simulink model "motor_model"  (R2018b)
settings: Solver=VariableStepAuto  StartTime=0.0  StopTime=2  RelTol=1e-3
model workspace (MAT data in the model file):
  Ce = 0.1
  Cm = 0.1
  Jsumm = 0.00025
  Kf = 0.1
  L = 0.0001
  R = 0.52
  U = 13.5
  poles = 8
libraries: simulink x2
settings Model: Creator=Sainquake  LastModifiedBy=Sainquake

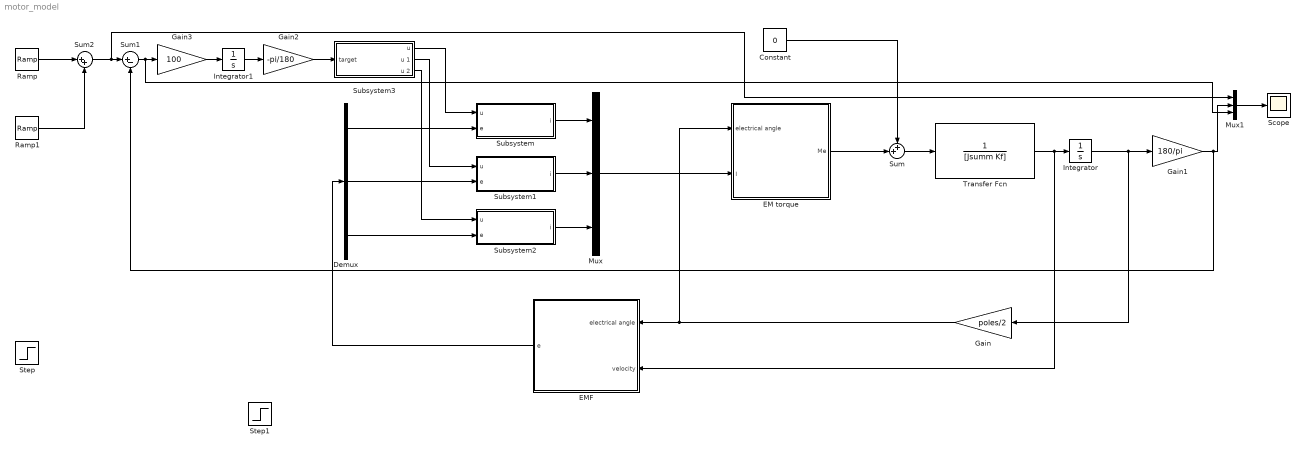
== system motor_model ==
  Constant : Constant  Value=0
  Demux : Demux  Outputs=3
  EM torque : Subsystem
  EMF : Subsystem
  Gain : Gain  Gain=poles/2
  Gain1 : Gain  Gain=180/pi
  Gain2 : Gain  Gain=-pi/180
  Gain3 : Gain  Gain=100
  Integrator : Integrator
  Integrator1 : Integrator
  Mux : Mux  Inputs=3
  Mux1 : Mux  Inputs=3
  Ramp : simulink/Sources/Ramp  slope=90/0.6  start=0  InitialOutput=0
  Ramp1 : simulink/Sources/Ramp  slope=-90/0.6  start=0.6  InitialOutput=0
  Scope : Scope
  Step : Step  Time=10  After=10  SampleTime=0
  Step1 : Step  SampleTime=0
  Subsystem : Subsystem
  Subsystem1 : Subsystem
  Subsystem2 : Subsystem
  Subsystem3 : Subsystem
  Sum : Sum  Inputs=++|
  Sum1 : Sum  Inputs=|+-
  Sum2 : Sum  Inputs=|++
  Transfer Fcn : TransferFcn  Denominator=[Jsumm Kf]
  wires:
  Subsystem/1(i) -> Mux/1
  Subsystem2/1(i) -> Mux/3
  Subsystem1/1(i) -> Mux/2
  Mux/1 -> EM torque/2(I)
  Demux/1 -> Subsystem/2("e ")
  Demux/2 -> Subsystem1/2("e ")
  Demux/3 -> Subsystem2/2("e ")
  EMF/1(e) -> Demux/1
  EM torque/1(Me) -> Sum/2
  Constant/1 -> Sum/1
  Sum/1 -> Transfer Fcn/1
  Transfer Fcn/1 -> EMF/2(velocity), Integrator/1
  Integrator/1 -> Gain1/1, Gain/1
  Gain/1 -> EM torque/1(electrical angle), EMF/1(electrical angle)
  Subsystem3/1("u ") -> Subsystem/1(u)
  Subsystem3/2(u 1) -> Subsystem1/1(u)
  Subsystem3/3(u 2) -> Subsystem2/1(u)
  Gain2/1 -> Subsystem3/1(target)
  Mux1/1 -> Scope/1
  Gain1/1 -> Mux1/2, Sum1/2
  Sum2/1 -> Mux1/1, Sum1/1
  Integrator1/1 -> Gain2/1
  Gain3/1 -> Integrator1/1
  Ramp/1 -> Sum2/1
  Ramp1/1 -> Sum2/2
  Sum1/1 -> Mux1/3, Gain3/1

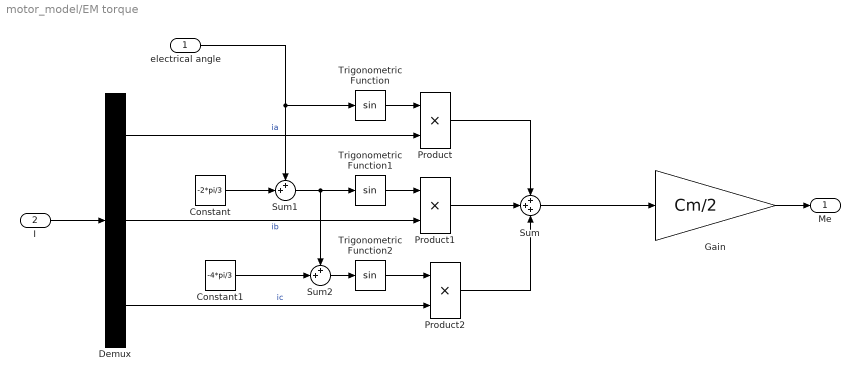
== system motor_model/EM torque ==
  electrical angle : Inport
  I : Inport  Port=2
  Constant : Constant  Value=-2*pi/3
  Constant1 : Constant  Value=-4*pi/3
  Demux : Demux  Outputs=3
  Gain : Gain  Gain=Cm/2
  Product : Product
  Product1 : Product
  Product2 : Product
  Sum : Sum  Inputs=+++
  Sum1 : Sum  Inputs=++|
  Sum2 : Sum  Inputs=++|
  Trigonometric Function : Trigonometry
  Trigonometric Function1 : Trigonometry
  Trigonometric Function2 : Trigonometry
  Me : Outport
  wires:
  Trigonometric Function/1 -> Product/1
  Product/1 -> Sum/1
  Sum/1 -> Gain/1
  Gain/1 -> Me/1
  Demux/1 -> Product/2  "ia"
  Trigonometric Function1/1 -> Product1/1
  Demux/2 -> Product1/2  "ib"
  Trigonometric Function2/1 -> Product2/1
  Demux/3 -> Product2/2  "ic"
  Product2/1 -> Sum/3
  Product1/1 -> Sum/2
  I/1 -> Demux/1
  Sum1/1 -> Sum2/1, Trigonometric Function1/1
  Constant/1 -> Sum1/2
  electrical angle/1 -> Trigonometric Function/1, Sum1/1
  Constant1/1 -> Sum2/2
  Sum2/1 -> Trigonometric Function2/1

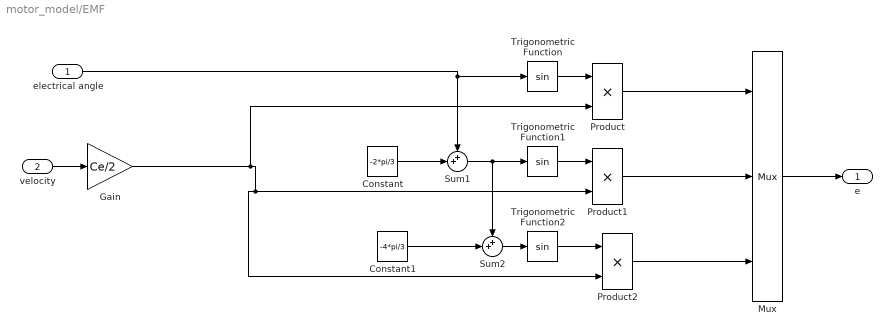
== system motor_model/EMF ==
  electrical angle : Inport
  velocity : Inport  Port=2
  Constant : Constant  Value=-2*pi/3
  Constant1 : Constant  Value=-4*pi/3
  Gain : Gain  Gain=Ce/2
  Mux : Mux  Inputs=3
  Product : Product
  Product1 : Product
  Product2 : Product
  Sum1 : Sum  Inputs=++|
  Sum2 : Sum  Inputs=++|
  Trigonometric Function : Trigonometry
  Trigonometric Function1 : Trigonometry
  Trigonometric Function2 : Trigonometry
  e : Outport
  wires:
  Trigonometric Function/1 -> Product/1
  Trigonometric Function1/1 -> Product1/1
  Trigonometric Function2/1 -> Product2/1
  Gain/1 -> Product2/2, Product1/2, Product/2
  Sum1/1 -> Sum2/1, Trigonometric Function1/1
  Constant/1 -> Sum1/2
  electrical angle/1 -> Trigonometric Function/1, Sum1/1
  Constant1/1 -> Sum2/2
  Sum2/1 -> Trigonometric Function2/1
  Mux/1 -> e/1
  velocity/1 -> Gain/1
  Product/1 -> Mux/1
  Product1/1 -> Mux/2
  Product2/1 -> Mux/3

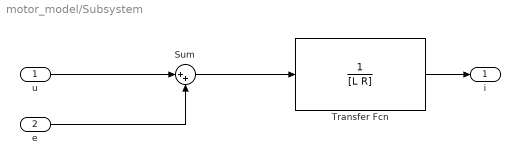
== system motor_model/Subsystem ==
  u : Inport
  "e " : Inport  Port=2
  Sum : Sum  Inputs=|++
  Transfer Fcn : TransferFcn  Denominator=[L R]
  i : Outport
  wires:
  u/1 -> Sum/1
  Transfer Fcn/1 -> i/1
  Sum/1 -> Transfer Fcn/1
  "e "/1 -> Sum/2

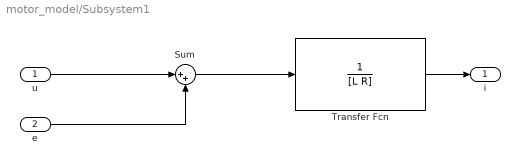
== system motor_model/Subsystem1 ==
  u : Inport
  "e " : Inport  Port=2
  Sum : Sum  Inputs=|++
  Transfer Fcn : TransferFcn  Denominator=[L R]
  i : Outport
  wires:
  u/1 -> Sum/1
  Transfer Fcn/1 -> i/1
  Sum/1 -> Transfer Fcn/1
  "e "/1 -> Sum/2

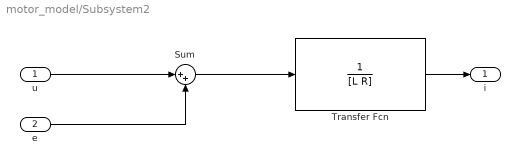
== system motor_model/Subsystem2 ==
  u : Inport
  "e " : Inport  Port=2
  Sum : Sum  Inputs=|++
  Transfer Fcn : TransferFcn  Denominator=[L R]
  i : Outport
  wires:
  u/1 -> Sum/1
  Transfer Fcn/1 -> i/1
  Sum/1 -> Transfer Fcn/1
  "e "/1 -> Sum/2

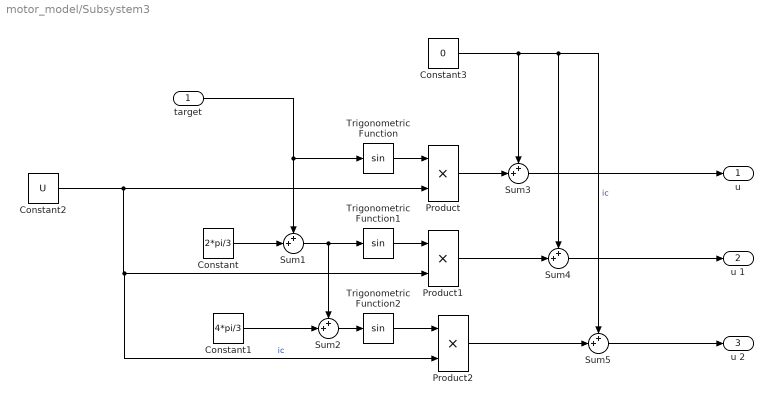
== system motor_model/Subsystem3 ==
  target : Inport
  Constant : Constant  Value=2*pi/3
  Constant1 : Constant  Value=4*pi/3
  Constant2 : Constant  Value=U
  Constant3 : Constant  Value=0
  Product : Product
  Product1 : Product
  Product2 : Product
  Sum{1..5} (5 alike) : Sum  Inputs=++|
  Trigonometric Function : Trigonometry
  Trigonometric Function1 : Trigonometry
  Trigonometric Function2 : Trigonometry
  "u " : Outport
  u 1 : Outport  Port=2
  u 2 : Outport  Port=3
  wires:
  Sum3/1 -> "u "/1
  target/1 -> Trigonometric Function/1, Sum1/1
  Trigonometric Function2/1 -> Product2/1
  Sum2/1 -> Trigonometric Function2/1
  Trigonometric Function1/1 -> Product1/1
  Constant2/1 -> Product/2, Product2/2, Product1/2  "ic"
  Constant1/1 -> Sum2/2
  Sum1/1 -> Sum2/1, Trigonometric Function1/1
  Constant/1 -> Sum1/2
  Trigonometric Function/1 -> Product/1
  Constant3/1 -> Sum5/1, Sum4/1, Sum3/1  "ic"
  Product/1 -> Sum3/2
  Product1/1 -> Sum4/2
  Product2/1 -> Sum5/2
  Sum5/1 -> u 2/1
  Sum4/1 -> u 1/1
